simulink model "S4"  (R2023b)
settings: Solver=FixedStepAuto  StartTime=0.0  StopTime=10  FixedStep=Step_T  RelTol=1e-3
values from neighbouring files (symbols this model uses):
  x_1_0 = 1    [P_sim.m]
  x_2_0 = -2    [P_sim.m]
settings Model: Creator=admin  LastModifiedBy=admin

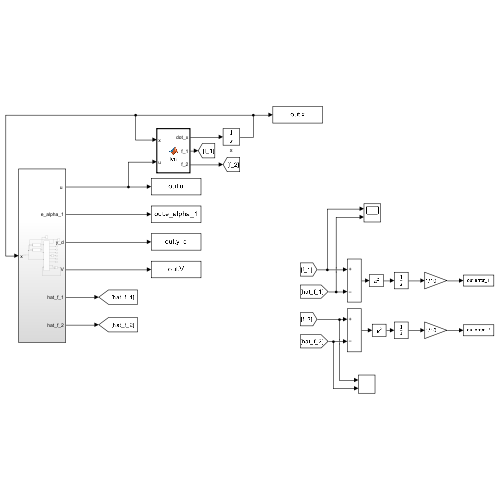
[thumbnail: Simulink's stored preview of the top-level diagram]
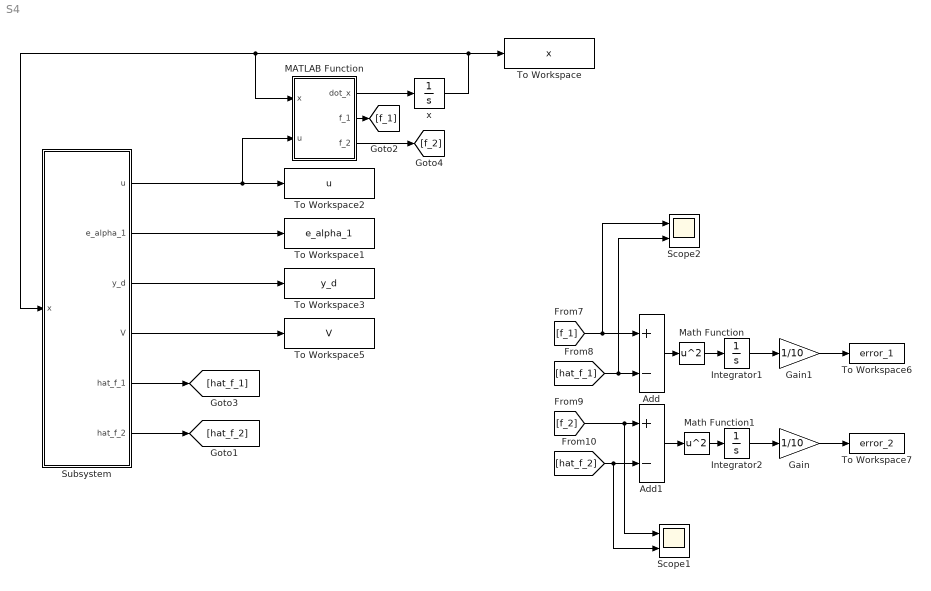
== system S4 ==
  Add : Sum  Inputs=+-
  Add1 : Sum  Inputs=+-
  Gain : Gain  Gain=1/10
  Gain1 : Gain  Gain=1/10
  Integrator1 : Integrator
  Integrator2 : Integrator
  MATLAB Function : MATLAB Function  TreatAsAtomicUnit=on
  Math Function : Math  Operator=square
  Math Function1 : Math  Operator=square
  Scope1 : Scope  NumInputPorts=2
  Scope2 : Scope  NumInputPorts=2
  Subsystem : Subsystem
  To Workspace : ToWorkspace  VariableName=x  SaveFormat=Timeseries  SampleTime=-1
  To Workspace1 : ToWorkspace  VariableName=e_alpha_1  SaveFormat=Timeseries  SampleTime=-1
  To Workspace2 : ToWorkspace  VariableName=u  SaveFormat=Timeseries  SampleTime=-1
  To Workspace3 : ToWorkspace  VariableName=y_d  SaveFormat=Timeseries  SampleTime=-1
  To Workspace5 : ToWorkspace  VariableName=V  SaveFormat=Timeseries  SampleTime=-1
  To Workspace6 : ToWorkspace  VariableName=error_1  SaveFormat=Timeseries  SampleTime=-1
  To Workspace7 : ToWorkspace  VariableName=error_2  SaveFormat=Timeseries  SampleTime=-1
  x : Integrator  InitialCondition=[x_1_0;x_2_0]
  wires:
  MATLAB Function/1(dot_x) -> x/1
  x/1 -> To Workspace/1, Subsystem/1(x), MATLAB Function/1(x)
  Subsystem/1("u ") -> MATLAB Function/2(u), To Workspace2/1
  Subsystem/2(e_alpha_1) -> To Workspace1/1
  Subsystem/3(y_d) -> To Workspace3/1
  Subsystem/4(V) -> To Workspace5/1
  Subsystem/5(hat_f_1) -> [hat_f_1]
  Subsystem/6(hat_f_2) -> [hat_f_2]
  MATLAB Function/2(f_1) -> [f_1]
  MATLAB Function/3(f_2) -> [f_2]
  Integrator1/1 -> Gain1/1
  Add/1 -> Math Function/1
  Add1/1 -> Math Function1/1
  [f_2] -> Scope1/1, Add1/1
  Integrator2/1 -> Gain/1
  Gain1/1 -> To Workspace6/1
  Math Function1/1 -> Integrator2/1
  [hat_f_2] -> Scope1/2, Add1/2
  [hat_f_1] -> Scope2/2, Add/2
  Math Function/1 -> Integrator1/1
  [f_1] -> Scope2/1, Add/1
  Gain/1 -> To Workspace7/1

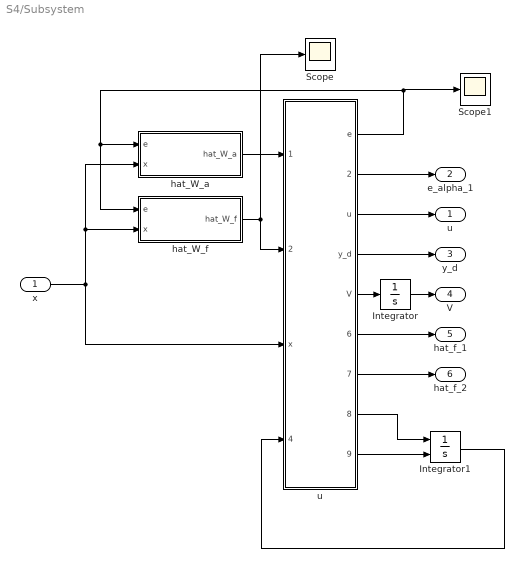
== system S4/Subsystem ==
  x : Inport
  Integrator : Integrator
  Integrator1 : Integrator  InitialConditionSource=external
  Scope : Scope
  Scope1 : Scope
  hat_W_a : Subsystem
  hat_W_f : Subsystem
  u : MATLAB Function  TreatAsAtomicUnit=on
  "u " : Outport
  e_alpha_1 : Outport  Port=2
  y_d : Outport  Port=3
  V : Outport  Port=4
  hat_f_1 : Outport  Port=5
  hat_f_2 : Outport  Port=6
  wires:
  u/3(u) -> "u "/1
  u/1(e) -> Scope1/1, hat_W_f/1(e), hat_W_a/1(e)
  u/4(y_d) -> y_d/1
  hat_W_f/1(hat_W_f) -> Scope/1, u/2(hat_W_f)
  hat_W_a/1(hat_W_a) -> u/1(hat_W_a)
  x/1 -> hat_W_a/2(x), hat_W_f/2(x), u/3(x)
  Integrator/1 -> V/1
  u/5(V) -> Integrator/1
  u/8(dot_alpha_1_d) -> Integrator1/1
  Integrator1/1 -> u/4(alpha_1_d)
  u/9(alpha_1) -> Integrator1/2
  u/2(e_alpha_1) -> e_alpha_1/1
  u/6(hat_f_1) -> hat_f_1/1
  u/7(hat_f_2) -> hat_f_2/1

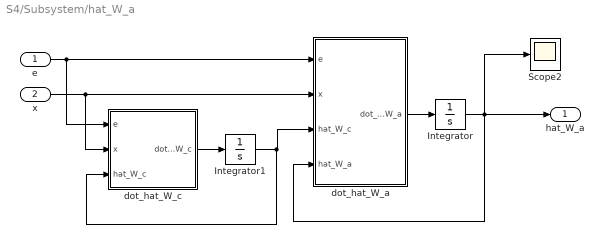
== system S4/Subsystem/hat_W_a ==
  e : Inport
  x : Inport  Port=2
  Integrator : Integrator  InitialCondition=0.3
  Integrator1 : Integrator  InitialCondition=-0.2
  Scope2 : Scope
  dot_hat_W_a : MATLAB Function  TreatAsAtomicUnit=on
  dot_hat_W_c : MATLAB Function  TreatAsAtomicUnit=on
  hat_W_a : Outport
  wires:
  dot_hat_W_a/1(dot_hat_W_a) -> Integrator/1
  Integrator/1 -> Scope2/1, dot_hat_W_a/4(hat_W_a), hat_W_a/1
  e/1 -> dot_hat_W_a/1(e), dot_hat_W_c/1(e)
  x/1 -> dot_hat_W_a/2(x), dot_hat_W_c/2(x)
  dot_hat_W_c/1(dot_hat_W_c) -> Integrator1/1
  Integrator1/1 -> dot_hat_W_c/3(hat_W_c), dot_hat_W_a/3(hat_W_c)

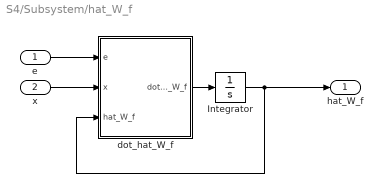
== system S4/Subsystem/hat_W_f ==
  e : Inport
  x : Inport  Port=2
  Integrator : Integrator  InitialCondition=0.1
  dot_hat_W_f : MATLAB Function  TreatAsAtomicUnit=on
  hat_W_f : Outport
  wires:
  dot_hat_W_f/1(dot_hat_W_f) -> Integrator/1
  Integrator/1 -> dot_hat_W_f/3(hat_W_f), hat_W_f/1
  e/1 -> dot_hat_W_f/1(e)
  x/1 -> dot_hat_W_f/2(x)

== matlab function S4/Subsystem/u ==
  data: e output size=[2,1]; e_alpha_1 output; hat_W_a input; hat_W_f input; x input size=[2,1]; u output; y_d output size=1; V output size=1; hat_f_1 output; hat_f_2 output; dot_alpha_1_d output; alpha_1 output; alpha_1_d input
function [e,e_alpha_1, u,y_d,V,hat_f_1,hat_f_2,dot_alpha_1_d,alpha_1]  = fcn(hat_W_a,hat_W_f,x,alpha_1_d)

y_d = 0;
dot_y_d = 0;

lambda_1 = 20;
lambda_2 = 20;
omega_1 = 0.005;

x_1 = x(1);
x_2 = x(2);

hat_W_a_1 = hat_W_a(:,1);
hat_W_a_2 = hat_W_a(:,2);

hat_W_f_1 = hat_W_f(:,1);
hat_W_f_2 = hat_W_f(:,2);

%% 第一阶
e_1 = x_1 - y_d;

S_f1 = RBF_based(x_1);
S_j1 = RBF_based([x_1;e_1]);

alpha_1 = -lambda_1*e_1-hat_W_f_1'*S_f1-hat_W_a_1'*S_j1+dot_y_d;
 
%% 第二阶
e_2 = x_2 - alpha_1;

S_f2 = RBF_based([x_1;x_2]);
S_j2 = RBF_based([x_1;x_2;e_2]);

dot_alpha_1_d = -(1/omega_1)*(alpha_1_d-alpha_1);
u = -lambda_2*e_2-hat_W_f_2'*S_f2-hat_W_a_2'*S_j2+dot_alpha_1_d;

e_alpha_1 = alpha_1_d-alpha_1;

e = [e_1;e_2];

V = e_1^2+u^2;
hat_f_1=hat_W_f_1'*S_f1;
hat_f_2=hat_W_f_2'*S_f2;

== matlab function S4/MATLAB Function ==
  data: x input; dot_x output; u input; pam parameter; f_1 output; f_2 output
function [dot_x,f_1,f_2]  = fcn(x,u,pam)

x_1 = x(1);
x_2 = x(2);

dot_x_1 = x_2-(1/pam.beta_1-pam.rho_1+sqrt(2))*x_1+cos(x_1);
dot_x_2 = u+sqrt(5)*x_1-(1/pam.beta_2-pam.rho_2)*x_2+sqrt(2)*sin(x_1)*cos(x_2);

dot_x = [dot_x_1;dot_x_2];
f_1 = -(1/pam.beta_1-pam.rho_1+sqrt(2))*x_1+cos(x_1);
f_2 = sqrt(5)*x_1-(1/pam.beta_2-pam.rho_2)*x_2+sqrt(2)*sin(x_1)*cos(x_2);

== matlab function S4/Subsystem/hat_W_f/dot_hat_W_f ==
  data: e input; x input; dot_hat_W_f output size=[24,2]; hat_W_f input
function dot_hat_W_f = fcn(e,x,hat_W_f)

x_1 = x(1);
x_2 = x(2);

e_1 = e(1);
e_2 = e(2);

hat_W_f_1 = hat_W_f(:,1);
hat_W_f_2 = hat_W_f(:,2);

%% 第一阶
S_f_1 = RBF_based(x_1);
dot_hat_W_f_1 = 2*(S_f_1*e_1-0.4*hat_W_f_1);
 
%% 第二阶
S_f_2 = RBF_based([x_1;x_2]);
dot_hat_W_f_2 = 2*(S_f_2*e_2-0.4*hat_W_f_2);


dot_hat_W_f = [dot_hat_W_f_1,dot_hat_W_f_2];

== matlab function S4/Subsystem/hat_W_a/dot_hat_W_a ==
  data: e input; x input; hat_W_c input; dot_hat_W_a output size=[24,2]; hat_W_a input
function dot_hat_W_a = fcn(e,x,hat_W_c,hat_W_a)

x_1 = x(1);
x_2 = x(2);

e_1 = e(1);
e_2 = e(2);

hat_W_a_1 = hat_W_a(:,1);
hat_W_a_2 = hat_W_a(:,2);

hat_W_c_1 = hat_W_c(:,1);
hat_W_c_2 = hat_W_c(:,2);

%% 第一阶
S_j1 = RBF_based([x_1;e_1]);
dot_hat_W_a_1 = -S_j1*S_j1'*(5*(hat_W_a_1-hat_W_c_1)+5*hat_W_c_1);
 
%% 第二阶
S_j2 = RBF_based([x_1;x_2;e_2]);
dot_hat_W_a_2 = -S_j2*S_j2'*(5*(hat_W_a_2-hat_W_c_2)+5*hat_W_c_2);


dot_hat_W_a = [dot_hat_W_a_1,dot_hat_W_a_2];

== matlab function S4/Subsystem/hat_W_a/dot_hat_W_c ==
  data: e input; x input; hat_W_c input size=[24,2]; dot_hat_W_c output
function dot_hat_W_c = fcn(e,x,hat_W_c)

x_1 = x(1);
x_2 = x(2);

e_1 = e(1);
e_2 = e(2);

hat_W_c_1 = hat_W_c(:,1);
hat_W_c_2 = hat_W_c(:,2);

%% 第一阶
S_j1 = RBF_based([x_1;e_1]);
dot_hat_W_c_1 = -5*(S_j1*S_j1')*hat_W_c_1;
 
%% 第二阶
S_j2 = RBF_based([x_1;x_2;e_2]);
dot_hat_W_c_2 = -5*(S_j2*S_j2')*hat_W_c_2;

dot_hat_W_c = [dot_hat_W_c_1,dot_hat_W_c_2];
